simulink model "mrefrobotarm_modified_previous_y_previous_u_previous_ref_pert_2"  (R2018b)
settings: Solver=FixedStepAuto  StartTime=0.0  StopTime=60  RelTol=1e-3  AbsTol=1e-6
undefined symbols (not defined in the file or in its folder): cc, options
libraries: neural x858, simulink x1
(part 14 of 32)

== system mrefrobotarm_modified_previous_y_previous_u_previous_ref_pert_2/m=0 sd=0.01/Layer 3/Delays 1 ==
  "p{3}" : Inport  PortDimensions=30
      mask Display: e = 0.06;c1 = [120 230 180]/255;c2 = ([120 230 180]+0)/(256+128);c3 = ([120 230 180]+128)/(256+128);patch([0 1 1 0],[0 0 1 1],c1);patch([0 1 1 1-e 1-e 0+e],[0 0 1 1-e 0+e 0+e],c2);patch([0 0 1 1-e 0+e 0+e],[0 1 1 1-e 1-e 0+e],c3);plot([0 1 1 0 0],[0 0 1 1 0]);
  mux : Mux  Inputs=1
      mask Display: e = 0.06;c1 = [120 150 230]/255;c2 = ([120 150 230]+0)/383;c3 = ([120 150 230]+128)/383;patch([0 1 1 0],[0 0 1 1],c1);patch([0 1 1 1-e 1-e 0+e],[0 0 1 1-e 0+e 0+e],c2);patch([0 0 1 1-e 0+e 0+e],[0 1 1 1-e 1-e 0+e],c3);plot([0 1 1 0 0],[0 0 1 1 0]);disp('Mux')
  "pd{3,2}" : Outport
      mask Display: e = 0.06;c1 = [120 230 180]/255;c2 = ([120 230 180]+0)/(256+128);c3 = ([120 230 180]+128)/(256+128);patch([0 1 1 0],[0 0 1 1],c1);patch([0 1 1 1-e 1-e 0+e],[0 0 1 1-e 0+e 0+e],c2);patch([0 0 1 1-e 0+e 0+e],[0 1 1 1-e 1-e 0+e],c3);plot([0 1 1 0 0],[0 0 1 1 0]);
  wires:
  "p{3}"/1 -> mux/1
  mux/1 -> "pd{3,2}"/1

== system mrefrobotarm_modified_previous_y_previous_u_previous_ref_pert_2/m=0 sd=0.01/Layer 3/LW{3,2} ==
  "ad{3,2}" : Inport  PortDimensions=30
      mask Display: e = 0.06;c1 = [120 230 180]/255;c2 = ([120 230 180]+0)/(256+128);c3 = ([120 230 180]+128)/(256+128);patch([0 1 1 0],[0 0 1 1],c1);patch([0 1 1 1-e 1-e 0+e],[0 0 1 1-e 0+e 0+e],c2);patch([0 0 1 1-e 0+e 0+e],[0 1 1 1-e 1-e 0+e],c3);plot([0 1 1 0 0],[0 0 1 1 0]);
  "IW{3,2}(1,:)'" : Constant  Value=[0.002729871880378900890484761276866265689022839069366455078125;-0.192793372477307212164987504365853965282440185546875;0.019007002077113754889836627626209519803524017333984375;0.1094735576049869207881926058689714409410953521728515625;-0.0344571917116396064795225129273603670299053192138671875;0.038374723582049762027335049197063199244439601898193359375;-0.271741639414177116318427351870923303067684173583984375;0.0219959957978727548011388392978915362618863582611083984375;0.0298221463111364611109355138296450604684650897979736328125;0.322074127211145644356093953319941647350788116455078125;0.13012962789399995511274710224824957549571990966796875;-0.00019342564852617015642988196333362793666310608386993408203125;0.043919430640314262304091386113213957287371158599853515625;-0.07079981267022698865343244278847123496234416961669921875;-0.039940672099975628450696518711993121542036533355712890625;-0.012214442964989628837013668771760421805083751678466796875;-0.434566982367647181018099900029483251273632049560546875;0.01100983664475223798573377820275709382258355617523193359375;0.013295194727414715030189285016604117117822170257568359375;0.00943231564172179563765308074607673916034400463104248046875;0.016511274981058310373782660462893545627593994140625;0.0083808882427890731003916613417459302581846714019775390625;-0.06728233732539042055709188616674509830772876739501953125;-0.0070167449523096288299672806942908209748566150665283203125;0.1945359442269654903778786092516384087502956390380859375;-0.10981910726153108759373111524837440811097621917724609375;-0.0295376597637224402870259609699132852256298065185546875;0.10283307654067570802158826381855760701000690460205078125;0.059639466058088001776393838326839613728225231170654296875;0.042842060625088405900751098442924558185040950775146484375]
      mask Display: e = 0.06;c1 = [120 150 230]/255;c2 = ([120 150 230]+0)/383;c3 = ([120 150 230]+128)/383;patch([0 1 1 0],[0 0 1 1],c1);patch([0 1 1 1-e 1-e 0+e],[0 0 1 1-e 0+e 0+e],c2);patch([0 0 1 1-e 0+e 0+e],[0 1 1 1-e 1-e 0+e],c3);plot([0 1 1 0 0],[0 0 1 1 0]);disp('weights');
  Mux : Mux  Inputs=1
      mask Display: e = 0.06;c1 = [120 150 230]/255;c2 = ([120 150 230]+0)/383;c3 = ([120 150 230]+128)/383;patch([0 1 1 0],[0 0 1 1],c1);patch([0 1 1 1-e 1-e 0+e],[0 0 1 1-e 0+e 0+e],c2);patch([0 0 1 1-e 0+e 0+e],[0 1 1 1-e 1-e 0+e],c3);plot([0 1 1 0 0],[0 0 1 1 0]);disp('Mux');
  dotprod1 : neural/Weight Functions/dotprod
  "lz{3,2}" : Outport
      mask Display: e = 0.06;c1 = [120 230 180]/255;c2 = ([120 230 180]+0)/(256+128);c3 = ([120 230 180]+128)/(256+128);patch([0 1 1 0],[0 0 1 1],c1);patch([0 1 1 1-e 1-e 0+e],[0 0 1 1-e 0+e 0+e],c2);patch([0 0 1 1-e 0+e 0+e],[0 1 1 1-e 1-e 0+e],c3);plot([0 1 1 0 0],[0 0 1 1 0]);
  wires:
  "IW{3,2}(1,:)'"/1 -> dotprod1/1
  "ad{3,2}"/1 -> dotprod1/2
  dotprod1/1 -> Mux/1
  Mux/1 -> "lz{3,2}"/1

== system mrefrobotarm_modified_previous_y_previous_u_previous_ref_pert_2/m=0 sd=0.1/Layer 1/Delays 1 ==
  "p{1}" : Inport  PortDimensions=10
      mask Display: e = 0.06;c1 = [120 230 180]/255;c2 = ([120 230 180]+0)/(256+128);c3 = ([120 230 180]+128)/(256+128);patch([0 1 1 0],[0 0 1 1],c1);patch([0 1 1 1-e 1-e 0+e],[0 0 1 1-e 0+e 0+e],c2);patch([0 0 1 1-e 0+e 0+e],[0 1 1 1-e 1-e 0+e],c3);plot([0 1 1 0 0],[0 0 1 1 0]);
  mux : Mux  Inputs=1
      mask Display: e = 0.06;c1 = [120 150 230]/255;c2 = ([120 150 230]+0)/383;c3 = ([120 150 230]+128)/383;patch([0 1 1 0],[0 0 1 1],c1);patch([0 1 1 1-e 1-e 0+e],[0 0 1 1-e 0+e 0+e],c2);patch([0 0 1 1-e 0+e 0+e],[0 1 1 1-e 1-e 0+e],c3);plot([0 1 1 0 0],[0 0 1 1 0]);disp('Mux')
  "pd{1,1}" : Outport
      mask Display: e = 0.06;c1 = [120 230 180]/255;c2 = ([120 230 180]+0)/(256+128);c3 = ([120 230 180]+128)/(256+128);patch([0 1 1 0],[0 0 1 1],c1);patch([0 1 1 1-e 1-e 0+e],[0 0 1 1-e 0+e 0+e],c2);patch([0 0 1 1-e 0+e 0+e],[0 1 1 1-e 1-e 0+e],c3);plot([0 1 1 0 0],[0 0 1 1 0]);
  wires:
  "p{1}"/1 -> mux/1
  mux/1 -> "pd{1,1}"/1

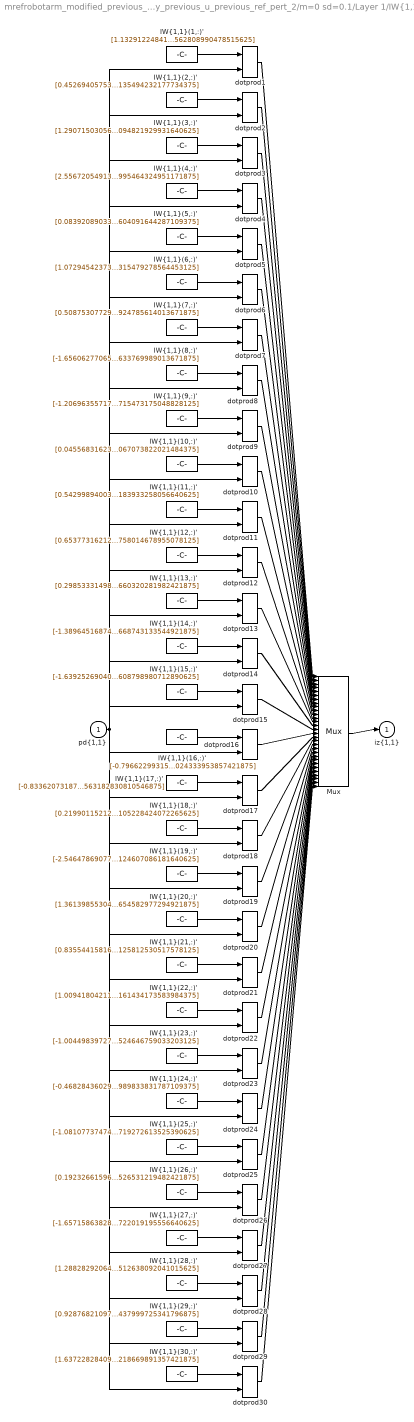
== system mrefrobotarm_modified_previous_y_previous_u_previous_ref_pert_2/m=0 sd=0.1/Layer 1/IW{1,1} ==
  "pd{1,1}" : Inport  PortDimensions=10
      mask Display: e = 0.06;c1 = [120 230 180]/255;c2 = ([120 230 180]+0)/(256+128);c3 = ([120 230 180]+128)/(256+128);patch([0 1 1 0],[0 0 1 1],c1);patch([0 1 1 1-e 1-e 0+e],[0 0 1 1-e 0+e 0+e],c2);patch([0 0 1 1-e 0+e 0+e],[0 1 1 1-e 1-e 0+e],c3);plot([0 1 1 0 0],[0 0 1 1 0]);
  "IW{1,1}(1,:)'" : Constant  Value=[1.132912248415559819392228746437467634677886962890625;-1.66311380994488278162179994978941977024078369140625;1.6836569926662872109801583064836449921131134033203125;-0.72192220583688004875710930718923918902873992919921875;0.1893688932828194448898528889912995509803295135498046875;-0.72187706282018548886725284319254569709300994873046875;-0.244996356013791827255232647075899876654148101806640625;-0.8003255307394396833586824868689291179180145263671875;0.85920037690395700824552704943926073610782623291015625;0.703707694441091380355146611691452562808990478515625]
      mask Display: e = 0.06;c1 = [120 150 230]/255;c2 = ([120 150 230]+0)/383;c3 = ([120 150 230]+128)/383;patch([0 1 1 0],[0 0 1 1],c1);patch([0 1 1 1-e 1-e 0+e],[0 0 1 1-e 0+e 0+e],c2);patch([0 0 1 1-e 0+e 0+e],[0 1 1 1-e 1-e 0+e],c3);plot([0 1 1 0 0],[0 0 1 1 0]);disp('Weights');
  "IW{1,1}(10,:)'" : Constant  Value=[0.04556831623344419213150757741459528915584087371826171875;-1.20856356098407413668383014737628400325775146484375;1.09655271159517742063371770200319588184356689453125;-1.2020275654665344422511452648905105888843536376953125;0.5891689284456680386625748724327422678470611572265625;-0.66781797039911106050880107432021759450435638427734375;0.92909816953891921631480954602011479437351226806640625;0.6734856783720146733429601226816885173320770263671875;-1.280385468531718640150529608945362269878387451171875;-1.3714212414356283797900459830998443067073822021484375]
      mask Display: e = 0.06;c1 = [120 150 230]/255;c2 = ([120 150 230]+0)/383;c3 = ([120 150 230]+128)/383;patch([0 1 1 0],[0 0 1 1],c1);patch([0 1 1 1-e 1-e 0+e],[0 0 1 1-e 0+e 0+e],c2);patch([0 0 1 1-e 0+e 0+e],[0 1 1 1-e 1-e 0+e],c3);plot([0 1 1 0 0],[0 0 1 1 0]);disp('Weights');
  "IW{1,1}(11,:)'" : Constant  Value=[0.5429989400329431337155483561218716204166412353515625;-1.3726786698952084808666995741077698767185211181640625;1.3447843857882892937283259016112424433231353759765625;0.06077100221745439234677377271509612910449504852294921875;0.14702327534578907286544335875078104436397552490234375;-0.9247467487885092651822560583241283893585205078125;1.214941057310911620703564040013588964939117431640625;0.51782811970024644754317932893172837793827056884765625;-0.5071720855890766710416528439964167773723602294921875;-0.84188455536436068715744340806850232183933258056640625]
      mask Display: e = 0.06;c1 = [120 150 230]/255;c2 = ([120 150 230]+0)/383;c3 = ([120 150 230]+128)/383;patch([0 1 1 0],[0 0 1 1],c1);patch([0 1 1 1-e 1-e 0+e],[0 0 1 1-e 0+e 0+e],c2);patch([0 0 1 1-e 0+e 0+e],[0 1 1 1-e 1-e 0+e],c3);plot([0 1 1 0 0],[0 0 1 1 0]);disp('Weights');
  "IW{1,1}(12,:)'" : Constant  Value=[0.6537731621292317552018857895745895802974700927734375;-0.6724403750684089242639629446784965693950653076171875;0.09800014716142928239417386748755234293639659881591796875;-0.0101106387101103749326380665252145263366401195526123046875;0.62476345499575847153295171665376983582973480224609375;-0.98464332271399535034817063205991871654987335205078125;0.29504906959603782734546939536812715232372283935546875;0.08629470772053095262155153477579005993902683258056640625;0.1016581340376631892308267879343475215137004852294921875;-0.63732167330842337538143738129292614758014678955078125]
      mask Display: e = 0.06;c1 = [120 150 230]/255;c2 = ([120 150 230]+0)/383;c3 = ([120 150 230]+128)/383;patch([0 1 1 0],[0 0 1 1],c1);patch([0 1 1 1-e 1-e 0+e],[0 0 1 1-e 0+e 0+e],c2);patch([0 0 1 1-e 0+e 0+e],[0 1 1 1-e 1-e 0+e],c3);plot([0 1 1 0 0],[0 0 1 1 0]);disp('Weights');
  "IW{1,1}(13,:)'" : Constant  Value=[0.29853331498265378574075157303013838827610015869140625;0.10168476545711895020485115992414648644626140594482421875;-0.478832017503906637312383054450037889182567596435546875;-0.345363443456295604594430415090755559504032135009765625;-0.365240575198647998700351990919443778693675994873046875;0.261408879776874325528979170485399663448333740234375;-0.126917798724279384803281800486729480326175689697265625;0.386500317068572074585830478099524043500423431396484375;0.813840320292881447272748118848539888858795166015625;-0.061249010278340447477329888670283253304660320281982421875]
      mask Display: e = 0.06;c1 = [120 150 230]/255;c2 = ([120 150 230]+0)/383;c3 = ([120 150 230]+128)/383;patch([0 1 1 0],[0 0 1 1],c1);patch([0 1 1 1-e 1-e 0+e],[0 0 1 1-e 0+e 0+e],c2);patch([0 0 1 1-e 0+e 0+e],[0 1 1 1-e 1-e 0+e],c3);plot([0 1 1 0 0],[0 0 1 1 0]);disp('Weights');
  "IW{1,1}(14,:)'" : Constant  Value=[-1.3896451687481945480584499819087795913219451904296875;2.15814199825849328817639616318047046661376953125;-1.2683298149542012733803630908369086682796478271484375;-0.11411191741998884252584645082606584765017032623291015625;-0.3155450540943876003296963972388766705989837646484375;0.1251853453557625339698233801755122840404510498046875;-0.00517304141358565679198466824573188205249607563018798828125;-0.64415172505282669579429466466535814106464385986328125;-0.64015313391352479666096542132436297833919525146484375;-0.259011561693888558988163595131481997668743133544921875]
      mask Display: e = 0.06;c1 = [120 150 230]/255;c2 = ([120 150 230]+0)/383;c3 = ([120 150 230]+128)/383;patch([0 1 1 0],[0 0 1 1],c1);patch([0 1 1 1-e 1-e 0+e],[0 0 1 1-e 0+e 0+e],c2);patch([0 0 1 1-e 0+e 0+e],[0 1 1 1-e 1-e 0+e],c3);plot([0 1 1 0 0],[0 0 1 1 0]);disp('Weights');
  "IW{1,1}(15,:)'" : Constant  Value=[-1.639252690409584101161044600303284823894500732421875;0.1935096092033950776478690158910467289388179779052734375;-0.5283754126046869004085237975232303142547607421875;0.57440826056501481655658380987006239593029022216796875;-0.229176783911712311780917161740944720804691314697265625;-1.46447525110886811461341494577936828136444091796875;0.65274531773674382417738115691463463008403778076171875;-0.50645703110697659621308730493183247745037078857421875;-1.0052356537245736856078792698099277913570404052734375;0.48612188066297401523030430325889028608798980712890625]
      mask Display: e = 0.06;c1 = [120 150 230]/255;c2 = ([120 150 230]+0)/383;c3 = ([120 150 230]+128)/383;patch([0 1 1 0],[0 0 1 1],c1);patch([0 1 1 1-e 1-e 0+e],[0 0 1 1-e 0+e 0+e],c2);patch([0 0 1 1-e 0+e 0+e],[0 1 1 1-e 1-e 0+e],c3);plot([0 1 1 0 0],[0 0 1 1 0]);disp('Weights');
  "IW{1,1}(16,:)'" : Constant  Value=[-0.79662299315886742068215653489460237324237823486328125;1.84598954255209957153738287161104381084442138671875;-0.94463712346467065827937403810210525989532470703125;-0.3956089994371831952690854450338520109653472900390625;-0.78376068618349925554156243379111401736736297607421875;-0.38177670775292316118765256760525517165660858154296875;0.61861305262131438542638761646230705082416534423828125;0.020921357743258151007381684394204057753086090087890625;0.4311848034144407648682317812927067279815673828125;-0.1757544230567029408529577949593658559024333953857421875]
      mask Display: e = 0.06;c1 = [120 150 230]/255;c2 = ([120 150 230]+0)/383;c3 = ([120 150 230]+128)/383;patch([0 1 1 0],[0 0 1 1],c1);patch([0 1 1 1-e 1-e 0+e],[0 0 1 1-e 0+e 0+e],c2);patch([0 0 1 1-e 0+e 0+e],[0 1 1 1-e 1-e 0+e],c3);plot([0 1 1 0 0],[0 0 1 1 0]);disp('Weights');
  "IW{1,1}(17,:)'" : Constant  Value=[-0.8336207318746462480163472719141282141208648681640625;0.72618402235620649332048515134374611079692840576171875;-0.53036297580617819402704071762855164706707000732421875;0.64140942781517551463110748954932205379009246826171875;-0.0221842617501962803550075165048838243819773197174072265625;-0.024558325479927707590821484018306364305317401885986328125;0.29991464523139754749792018628795631229877471923828125;0.16921995587321048137852130821556784212589263916015625;-0.90896451623632634753136017025099135935306549072265625;-0.1841664914636124972258102161504211835563182830810546875]
      mask Display: e = 0.06;c1 = [120 150 230]/255;c2 = ([120 150 230]+0)/383;c3 = ([120 150 230]+128)/383;patch([0 1 1 0],[0 0 1 1],c1);patch([0 1 1 1-e 1-e 0+e],[0 0 1 1-e 0+e 0+e],c2);patch([0 0 1 1-e 0+e 0+e],[0 1 1 1-e 1-e 0+e],c3);plot([0 1 1 0 0],[0 0 1 1 0]);disp('Weights');
  "IW{1,1}(18,:)'" : Constant  Value=[0.219901152121808662887048058109940029680728912353515625;-0.09076825686005864091132622206714586354792118072509765625;-0.339186564269195633958275948316440917551517486572265625;-0.502276581787442832904844181030057370662689208984375;-0.413214937935847126393440476022078655660152435302734375;0.406702355871940646192541635173256509006023406982421875;0.015662906329028440655104503775874036364257335662841796875;-0.5416305832111605322864988920628093183040618896484375;0.314207839020848311850642176068504340946674346923828125;0.021790223956706523955606513709426508285105228424072265625]
      mask Display: e = 0.06;c1 = [120 150 230]/255;c2 = ([120 150 230]+0)/383;c3 = ([120 150 230]+128)/383;patch([0 1 1 0],[0 0 1 1],c1);patch([0 1 1 1-e 1-e 0+e],[0 0 1 1-e 0+e 0+e],c2);patch([0 0 1 1-e 0+e 0+e],[0 1 1 1-e 1-e 0+e],c3);plot([0 1 1 0 0],[0 0 1 1 0]);disp('Weights');
  "IW{1,1}(19,:)'" : Constant  Value=[-2.54647869077617716726535945781506597995758056640625;2.074022456073995268610588027513585984706878662109375;-1.264725581662340392341548067633993923664093017578125;0.269992056926158074947608156435308046638965606689453125;0.67791205426768907926771134953014552593231201171875;1.08945288321787092655767992255277931690216064453125;-0.225879558387034384825398092289105989038944244384765625;-0.8743718013102685926440926778013817965984344482421875;1.313495208741327413548560798517428338527679443359375;0.88931998964906144866660042680450715124607086181640625]
      mask Display: e = 0.06;c1 = [120 150 230]/255;c2 = ([120 150 230]+0)/383;c3 = ([120 150 230]+128)/383;patch([0 1 1 0],[0 0 1 1],c1);patch([0 1 1 1-e 1-e 0+e],[0 0 1 1-e 0+e 0+e],c2);patch([0 0 1 1-e 0+e 0+e],[0 1 1 1-e 1-e 0+e],c3);plot([0 1 1 0 0],[0 0 1 1 0]);disp('Weights');
  "IW{1,1}(2,:)'" : Constant  Value=[0.45269405753099623002100315716234035789966583251953125;-1.3819854543589837891914839929086156189441680908203125;1.4394656881736762610302093889913521707057952880859375;-0.498626309305983339559276146246702410280704498291015625;-0.414204872178560890016996154372463934123516082763671875;1.55952109847031028522224005428142845630645751953125;-0.56120044368516330823837279240251518785953521728515625;-0.281840967673469833254529248733888380229473114013671875;3.50820378995669113209032730082981288433074951171875;2.044493088024915916633972301497124135494232177734375]
      mask Display: e = 0.06;c1 = [120 150 230]/255;c2 = ([120 150 230]+0)/383;c3 = ([120 150 230]+128)/383;patch([0 1 1 0],[0 0 1 1],c1);patch([0 1 1 1-e 1-e 0+e],[0 0 1 1-e 0+e 0+e],c2);patch([0 0 1 1-e 0+e 0+e],[0 1 1 1-e 1-e 0+e],c3);plot([0 1 1 0 0],[0 0 1 1 0]);disp('Weights');
  "IW{1,1}(20,:)'" : Constant  Value=[1.361398553041379244632480549626052379608154296875;-1.3859070894705352028353217974654398858547210693359375;-0.400969251454327435535418544532149098813533782958984375;-0.427897979455180876851017046647029928863048553466796875;0.63437067973309779755908266452024690806865692138671875;0.334528713373865083102742801202111877501010894775390625;0.05397557593578884704843545705443830229341983795166015625;0.13660549295664325963883811709820292890071868896484375;1.049795083463204381502009709947742521762847900390625;-0.0200764131524870208245214797670996631495654582977294921875]
      mask Display: e = 0.06;c1 = [120 150 230]/255;c2 = ([120 150 230]+0)/383;c3 = ([120 150 230]+128)/383;patch([0 1 1 0],[0 0 1 1],c1);patch([0 1 1 1-e 1-e 0+e],[0 0 1 1-e 0+e 0+e],c2);patch([0 0 1 1-e 0+e 0+e],[0 1 1 1-e 1-e 0+e],c3);plot([0 1 1 0 0],[0 0 1 1 0]);disp('Weights');
  "IW{1,1}(21,:)'" : Constant  Value=[0.83554415816043192677398110390640795230865478515625;-0.75667157664683060147581272758543491363525390625;-0.05035462838145922381816177448854432441294193267822265625;-0.186509261977637230689452962906216271221637725830078125;0.1779164267290028467183304883292294107377529144287109375;-0.16737486559107284112002389520057477056980133056640625;-0.043842380630178291733844986310941749252378940582275390625;0.30516299405469571315308030534652061760425567626953125;-1.527210479319259572861255946918390691280364990234375;-0.5785736861187509294524033975903876125812530517578125]
      mask Display: e = 0.06;c1 = [120 150 230]/255;c2 = ([120 150 230]+0)/383;c3 = ([120 150 230]+128)/383;patch([0 1 1 0],[0 0 1 1],c1);patch([0 1 1 1-e 1-e 0+e],[0 0 1 1-e 0+e 0+e],c2);patch([0 0 1 1-e 0+e 0+e],[0 1 1 1-e 1-e 0+e],c3);plot([0 1 1 0 0],[0 0 1 1 0]);disp('Weights');
  "IW{1,1}(22,:)'" : Constant  Value=[1.00941804211583718853262325865216553211212158203125;-1.2261900889778554191167359022074379026889801025390625;0.120851782045483469030244805253460071980953216552734375;0.32676568345732548426241237393696792423725128173828125;-0.52634117539310398825591619242914021015167236328125;1.1012958159960113402320303066517226397991180419921875;-0.5060253977059598895493763848207890987396240234375;-0.39813348380348656530003381703863851726055145263671875;1.8147553018736901631058344719349406659603118896484375;1.4870405850798051883288053431897424161434173583984375]
      mask Display: e = 0.06;c1 = [120 150 230]/255;c2 = ([120 150 230]+0)/383;c3 = ([120 150 230]+128)/383;patch([0 1 1 0],[0 0 1 1],c1);patch([0 1 1 1-e 1-e 0+e],[0 0 1 1-e 0+e 0+e],c2);patch([0 0 1 1-e 0+e 0+e],[0 1 1 1-e 1-e 0+e],c3);plot([0 1 1 0 0],[0 0 1 1 0]);disp('Weights');
  "IW{1,1}(23,:)'" : Constant  Value=[-1.0044983972705108232759130260092206299304962158203125;0.1873298225454137211354321834733127616345882415771484375;-0.54804213617540142866602081994642503559589385986328125;-0.70042673178915515475040365345194004476070404052734375;-0.023415375354162000498536855275233392603695392608642578125;-0.95501032317440992525092724463320337235927581787109375;1.0022110698728763367171268328092992305755615234375;-0.76991655197060937521058576749055646359920501708984375;-1.02462948914607299144563512527383863925933837890625;-1.4760810948051397151203900648397393524646759033203125]
      mask Display: e = 0.06;c1 = [120 150 230]/255;c2 = ([120 150 230]+0)/383;c3 = ([120 150 230]+128)/383;patch([0 1 1 0],[0 0 1 1],c1);patch([0 1 1 1-e 1-e 0+e],[0 0 1 1-e 0+e 0+e],c2);patch([0 0 1 1-e 0+e 0+e],[0 1 1 1-e 1-e 0+e],c3);plot([0 1 1 0 0],[0 0 1 1 0]);disp('Weights');
  "IW{1,1}(24,:)'" : Constant  Value=[-0.468284360290036671958802116932929493486881256103515625;1.0621707027343048057588248411775566637516021728515625;-0.91950497784860119043770509961177594959735870361328125;0.050729086990261358647291700663117808289825916290283203125;0.09401277611720904037184709522989578545093536376953125;-0.5526691859768873005265277242870070040225982666015625;0.6698966360936118302760178266908042132854461669921875;-0.1567729090403978398082784906364395283162593841552734375;0.264933900169632863264013167281518690288066864013671875;-0.447551825822690485523480674601159989833831787109375]
      mask Display: e = 0.06;c1 = [120 150 230]/255;c2 = ([120 150 230]+0)/383;c3 = ([120 150 230]+128)/383;patch([0 1 1 0],[0 0 1 1],c1);patch([0 1 1 1-e 1-e 0+e],[0 0 1 1-e 0+e 0+e],c2);patch([0 0 1 1-e 0+e 0+e],[0 1 1 1-e 1-e 0+e],c3);plot([0 1 1 0 0],[0 0 1 1 0]);disp('Weights');
  "IW{1,1}(25,:)'" : Constant  Value=[-1.081077374740320617974020933615975081920623779296875;0.64279083661811375893790909685776568949222564697265625;-0.267842395764306850924896252763574011623859405517578125;0.7450897607842363878916103203664533793926239013671875;0.82627356030284893062543005726183764636516571044921875;-0.39195769077825470816378583549521863460540771484375;-0.202015501963519417127912447540438733994960784912109375;0.89916101439714213316989344093599356710910797119140625;-0.8301541281567679231301326581160537898540496826171875;-0.416799917133972963600996308741741813719272613525390625]
      mask Display: e = 0.06;c1 = [120 150 230]/255;c2 = ([120 150 230]+0)/383;c3 = ([120 150 230]+128)/383;patch([0 1 1 0],[0 0 1 1],c1);patch([0 1 1 1-e 1-e 0+e],[0 0 1 1-e 0+e 0+e],c2);patch([0 0 1 1-e 0+e 0+e],[0 1 1 1-e 1-e 0+e],c3);plot([0 1 1 0 0],[0 0 1 1 0]);disp('Weights');
  "IW{1,1}(26,:)'" : Constant  Value=[0.1923266159612029568837243687084992416203022003173828125;-0.80992252631693961717473939643241465091705322265625;-0.14493676196781934972790395477204583585262298583984375;-1.1229707457292572581053491376223973929882049560546875;-0.54252404045220148365302748061367310583591461181640625;-1.06886334868473031889379853964783251285552978515625;0.9948315499383790783127778922789730131626129150390625;0.152465655384979414943558140294044278562068939208984375;-0.68998166028190721643653660066775046288967132568359375;-1.4428166074457855483359480786020867526531219482421875]
      mask Display: e = 0.06;c1 = [120 150 230]/255;c2 = ([120 150 230]+0)/383;c3 = ([120 150 230]+128)/383;patch([0 1 1 0],[0 0 1 1],c1);patch([0 1 1 1-e 1-e 0+e],[0 0 1 1-e 0+e 0+e],c2);patch([0 0 1 1-e 0+e 0+e],[0 1 1 1-e 1-e 0+e],c3);plot([0 1 1 0 0],[0 0 1 1 0]);disp('Weights');
  "IW{1,1}(27,:)'" : Constant  Value=[-1.6571586382832157458011579365120269358158111572265625;2.86298728904135391104546215501613914966583251953125;-0.7213543770211312544660131607088260352611541748046875;0.301232704656333172277271614802884869277477264404296875;-0.016745756818622899164683559547484037466347217559814453125;-0.82008705446743979106116739785647951066493988037109375;0.65578457676010992738468985407962463796138763427734375;-0.68340853893493924697821739755454473197460174560546875;0.1911644525940358885218728346444549970328807830810546875;-0.0288623922702351022595568252882003434933722019195556640625]
      mask Display: e = 0.06;c1 = [120 150 230]/255;c2 = ([120 150 230]+0)/383;c3 = ([120 150 230]+128)/383;patch([0 1 1 0],[0 0 1 1],c1);patch([0 1 1 1-e 1-e 0+e],[0 0 1 1-e 0+e 0+e],c2);patch([0 0 1 1-e 0+e 0+e],[0 1 1 1-e 1-e 0+e],c3);plot([0 1 1 0 0],[0 0 1 1 0]);disp('Weights');
  "IW{1,1}(28,:)'" : Constant  Value=[1.2882829206406238853332979488186538219451904296875;-0.62425953029952607753472193508059717714786529541015625;-0.59190041246323155110786728982930071651935577392578125;0.53647381032516161525336428894661366939544677734375;0.42978817559882898091672132068197242915630340576171875;0.70153054187913921335706390891573391854763031005859375;-0.458324045413930847292505177392740733921527862548828125;-0.50252223793030947884830084149143658578395843505859375;-0.91259450157277643977948855535942129790782928466796875;-0.130631405538267186816625553547055460512638092041015625]
      mask Display: e = 0.06;c1 = [120 150 230]/255;c2 = ([120 150 230]+0)/383;c3 = ([120 150 230]+128)/383;patch([0 1 1 0],[0 0 1 1],c1);patch([0 1 1 1-e 1-e 0+e],[0 0 1 1-e 0+e 0+e],c2);patch([0 0 1 1-e 0+e 0+e],[0 1 1 1-e 1-e 0+e],c3);plot([0 1 1 0 0],[0 0 1 1 0]);disp('Weights');
  "IW{1,1}(29,:)'" : Constant  Value=[0.92876821097719874931186723188147880136966705322265625;-0.316191487680865190856849267220241017639636993408203125;-0.9663850736922203754630800176528282463550567626953125;-0.68849439879813878473413524261559359729290008544921875;-0.429687888689719910129127811160287819802761077880859375;0.289887888189278408734850245309644378721714019775390625;1.278858531308505686041598892188630998134613037109375;-0.8698389651444429215843001657049171626567840576171875;1.0468948855574324863226820525596849620342254638671875;-0.1539409925282792801493059187123435549437999725341796875]
      mask Display: e = 0.06;c1 = [120 150 230]/255;c2 = ([120 150 230]+0)/383;c3 = ([120 150 230]+128)/383;patch([0 1 1 0],[0 0 1 1],c1);patch([0 1 1 1-e 1-e 0+e],[0 0 1 1-e 0+e 0+e],c2);patch([0 0 1 1-e 0+e 0+e],[0 1 1 1-e 1-e 0+e],c3);plot([0 1 1 0 0],[0 0 1 1 0]);disp('Weights');
  "IW{1,1}(3,:)'" : Constant  Value=[1.2907150305671650780681147807626985013484954833984375;-1.5769416133466929164086423043045215308666229248046875;-0.66001303824557966404285025419085286557674407958984375;0.52837771369532327003781801977311260998249053955078125;0.521070941990531277809850507765077054500579833984375;-0.74814857171303950078566913362010382115840911865234375;1.02852301966715931058615751680918037891387939453125;-0.1321655342391363507914547881227917969226837158203125;-0.456989775756285798724576352469739504158496856689453125;-0.6231284026776793272262011669226922094821929931640625]
      mask Display: e = 0.06;c1 = [120 150 230]/255;c2 = ([120 150 230]+0)/383;c3 = ([120 150 230]+128)/383;patch([0 1 1 0],[0 0 1 1],c1);patch([0 1 1 1-e 1-e 0+e],[0 0 1 1-e 0+e 0+e],c2);patch([0 0 1 1-e 0+e 0+e],[0 1 1 1-e 1-e 0+e],c3);plot([0 1 1 0 0],[0 0 1 1 0]);disp('Weights');
  "IW{1,1}(30,:)'" : Constant  Value=[1.637228284090687768781435806886292994022369384765625;-1.846953752864070708028521039523184299468994140625;0.6806049332873114199315978112281300127506256103515625;-0.56541885127706914548895156258367933332920074462890625;-1.2699089669929273238579980898066423833370208740234375;1.86689761180617797009517744299955666065216064453125;-1.1232513546886908617494782447465695440769195556640625;0.1453674639014009006832139903053757734596729278564453125;1.0509840057341672814317234951886348426342010498046875;1.505179218361568427297925154562108218669891357421875]
      mask Display: e = 0.06;c1 = [120 150 230]/255;c2 = ([120 150 230]+0)/383;c3 = ([120 150 230]+128)/383;patch([0 1 1 0],[0 0 1 1],c1);patch([0 1 1 1-e 1-e 0+e],[0 0 1 1-e 0+e 0+e],c2);patch([0 0 1 1-e 0+e 0+e],[0 1 1 1-e 1-e 0+e],c3);plot([0 1 1 0 0],[0 0 1 1 0]);disp('Weights');
  "IW{1,1}(4,:)'" : Constant  Value=[2.556720549135189202161200228147208690643310546875;-3.258857965265137490717961554764769971370697021484375;1.1401735662930827519545573522918857634067535400390625;-0.527964829625254150613500314648263156414031982421875;1.9440738356444582368709461661637760698795318603515625;-0.7482336793844714950552088339463807642459869384765625;-0.3204906509866918273843339193263091146945953369140625;1.06815648950187647159282278153114020824432373046875;-0.0890878366209650607299153080020914785563945770263671875;-0.98332734514651221058301189259509555995464324951171875]
      mask Display: e = 0.06;c1 = [120 150 230]/255;c2 = ([120 150 230]+0)/383;c3 = ([120 150 230]+128)/383;patch([0 1 1 0],[0 0 1 1],c1);patch([0 1 1 1-e 1-e 0+e],[0 0 1 1-e 0+e 0+e],c2);patch([0 0 1 1-e 0+e 0+e],[0 1 1 1-e 1-e 0+e],c3);plot([0 1 1 0 0],[0 0 1 1 0]);disp('Weights');
  "IW{1,1}(5,:)'" : Constant  Value=[0.08392089033110028406525771060842089354991912841796875;-0.01076518165151564392079119869549685972742736339569091796875;-0.76431051909334024596631707026972435414791107177734375;0.005445241138962057976524722135991396498866379261016845703125;-1.113896888451066491398933067102916538715362548828125;1.1829549197050621689442095885169692337512969970703125;-0.1452638359721234173616011275953496806323528289794921875;0.09505325241205352104767456467016017995774745941162109375;0.824643225782639266441265135654248297214508056640625;1.148108113835907939659364274120889604091644287109375]
      mask Display: e = 0.06;c1 = [120 150 230]/255;c2 = ([120 150 230]+0)/383;c3 = ([120 150 230]+128)/383;patch([0 1 1 0],[0 0 1 1],c1);patch([0 1 1 1-e 1-e 0+e],[0 0 1 1-e 0+e 0+e],c2);patch([0 0 1 1-e 0+e 0+e],[0 1 1 1-e 1-e 0+e],c3);plot([0 1 1 0 0],[0 0 1 1 0]);disp('Weights');
  "IW{1,1}(6,:)'" : Constant  Value=[1.0729454237326871979263387402170337736606597900390625;-1.02897733435734739515510227647610008716583251953125;0.529513108661344933381087685120292007923126220703125;-0.160761617828738045954395374792511574923992156982421875;-0.255155535700625157868870473976130597293376922607421875;-0.4693729374857118497033070525503717362880706787109375;0.92985584320082781406568983584293164312839508056640625;-0.203429108007346759467992569625494070351123809814453125;0.0677569643726999848443171003964380361139774322509765625;-0.5436491628863440173091703400132246315479278564453125]
      mask Display: e = 0.06;c1 = [120 150 230]/255;c2 = ([120 150 230]+0)/383;c3 = ([120 150 230]+128)/383;patch([0 1 1 0],[0 0 1 1],c1);patch([0 1 1 1-e 1-e 0+e],[0 0 1 1-e 0+e 0+e],c2);patch([0 0 1 1-e 0+e 0+e],[0 1 1 1-e 1-e 0+e],c3);plot([0 1 1 0 0],[0 0 1 1 0]);disp('Weights');
  "IW{1,1}(7,:)'" : Constant  Value=[0.5087530772928250399900207412429153919219970703125;-0.72275590797490962824412008558283559978008270263671875;0.98703592833260522798610736572300083935260772705078125;0.0745257436909177173323115539460559375584125518798828125;-0.515275994488835209494936862029135227203369140625;0.408520690147010867576682358048856258392333984375;0.7049744986580306349566171775222755968570709228515625;-0.5187749998269481910284639525343663990497589111328125;-0.655588975122619377344790336792357265949249267578125;-1.192263238986935647290010820142924785614013671875]
      mask Display: e = 0.06;c1 = [120 150 230]/255;c2 = ([120 150 230]+0)/383;c3 = ([120 150 230]+128)/383;patch([0 1 1 0],[0 0 1 1],c1);patch([0 1 1 1-e 1-e 0+e],[0 0 1 1-e 0+e 0+e],c2);patch([0 0 1 1-e 0+e 0+e],[0 1 1 1-e 1-e 0+e],c3);plot([0 1 1 0 0],[0 0 1 1 0]);disp('Weights');
  "IW{1,1}(8,:)'" : Constant  Value=[-1.656062770656069549346511848852969706058502197265625;1.0799485487971907105020363815128803253173828125;1.07643846673486809351061310735531151294708251953125;-0.11388515890106561123662487489127670414745807647705078125;0.34417213396941293002129214073647744953632354736328125;-0.035461693978427459572611013527421164326369762420654296875;-1.3084703437418314653228890165337361395359039306640625;0.1805781658817567081332100542567786760628223419189453125;1.492291368578742893902244759374298155307769775390625;1.223695843846154929224212537519633769989013671875]
      mask Display: e = 0.06;c1 = [120 150 230]/255;c2 = ([120 150 230]+0)/383;c3 = ([120 150 230]+128)/383;patch([0 1 1 0],[0 0 1 1],c1);patch([0 1 1 1-e 1-e 0+e],[0 0 1 1-e 0+e 0+e],c2);patch([0 0 1 1-e 0+e 0+e],[0 1 1 1-e 1-e 0+e],c3);plot([0 1 1 0 0],[0 0 1 1 0]);disp('Weights');
  "IW{1,1}(9,:)'" : Constant  Value=[-1.2069635571783063898720911311102099716663360595703125;-0.1954715592676647684111657099492731504142284393310546875;2.2208001581531267021318853949196636676788330078125;-0.56222673478999263263489183373167179524898529052734375;1.2816598991110985661379118027980439364910125732421875;1.4310647588806173491349227333557792007923126220703125;-2.554919380782112892092072797822766005992889404296875;0.2336960307259200730900516873589367605745792388916015625;0.63656718069432993711842527773114852607250213623046875;1.1105605139442176199082723542232997715473175048828125]
      mask Display: e = 0.06;c1 = [120 150 230]/255;c2 = ([120 150 230]+0)/383;c3 = ([120 150 230]+128)/383;patch([0 1 1 0],[0 0 1 1],c1);patch([0 1 1 1-e 1-e 0+e],[0 0 1 1-e 0+e 0+e],c2);patch([0 0 1 1-e 0+e 0+e],[0 1 1 1-e 1-e 0+e],c3);plot([0 1 1 0 0],[0 0 1 1 0]);disp('Weights');
  Mux : Mux  Inputs=30
      mask Display: e = 0.06;c1 = [120 150 230]/255;c2 = ([120 150 230]+0)/383;c3 = ([120 150 230]+128)/383;patch([0 1 1 0],[0 0 1 1],c1);patch([0 1 1 1-e 1-e 0+e],[0 0 1 1-e 0+e 0+e],c2);patch([0 0 1 1-e 0+e 0+e],[0 1 1 1-e 1-e 0+e],c3);plot([0 1 1 0 0],[0 0 1 1 0]);disp('Mux');
  dotprod{1..30} (30 alike) : neural/Weight Functions/dotprod
  "iz{1,1}" : Outport
      mask Display: e = 0.06;c1 = [120 230 180]/255;c2 = ([120 230 180]+0)/(256+128);c3 = ([120 230 180]+128)/(256+128);patch([0 1 1 0],[0 0 1 1],c1);patch([0 1 1 1-e 1-e 0+e],[0 0 1 1-e 0+e 0+e],c2);patch([0 0 1 1-e 0+e 0+e],[0 1 1 1-e 1-e 0+e],c3);plot([0 1 1 0 0],[0 0 1 1 0]);
  wires:
  "IW{1,1}(1,:)'"/1 -> dotprod1/1
  "pd{1,1}"/1 -> dotprod1/2, dotprod2/2, dotprod3/2, dotprod4/2, dotprod5/2, dotprod6/2, dotprod7/2, dotprod8/2, dotprod9/2, dotprod10/2, dotprod11/2, dotprod12/2, dotprod13/2, dotprod14/2, dotprod15/2, dotprod16/2, dotprod17/2, dotprod18/2, dotprod19/2, dotprod20/2, dotprod21/2, dotprod22/2, dotprod23/2, dotprod24/2, dotprod25/2, dotprod26/2, dotprod27/2, dotprod28/2, dotprod29/2, dotprod30/2
  dotprod1/1 -> Mux/1
  "IW{1,1}(2,:)'"/1 -> dotprod2/1
  dotprod2/1 -> Mux/2
  "IW{1,1}(3,:)'"/1 -> dotprod3/1
  dotprod3/1 -> Mux/3
  "IW{1,1}(4,:)'"/1 -> dotprod4/1
  dotprod4/1 -> Mux/4
  "IW{1,1}(5,:)'"/1 -> dotprod5/1
  dotprod5/1 -> Mux/5
  "IW{1,1}(6,:)'"/1 -> dotprod6/1
  dotprod6/1 -> Mux/6
  "IW{1,1}(7,:)'"/1 -> dotprod7/1
  dotprod7/1 -> Mux/7
  "IW{1,1}(8,:)'"/1 -> dotprod8/1
  dotprod8/1 -> Mux/8
  "IW{1,1}(9,:)'"/1 -> dotprod9/1
  dotprod9/1 -> Mux/9
  "IW{1,1}(10,:)'"/1 -> dotprod10/1
  dotprod10/1 -> Mux/10
  "IW{1,1}(11,:)'"/1 -> dotprod11/1
  dotprod11/1 -> Mux/11
  "IW{1,1}(12,:)'"/1 -> dotprod12/1
  dotprod12/1 -> Mux/12
  "IW{1,1}(13,:)'"/1 -> dotprod13/1
  dotprod13/1 -> Mux/13
  "IW{1,1}(14,:)'"/1 -> dotprod14/1
  dotprod14/1 -> Mux/14
  "IW{1,1}(15,:)'"/1 -> dotprod15/1
  dotprod15/1 -> Mux/15
  "IW{1,1}(16,:)'"/1 -> dotprod16/1
  dotprod16/1 -> Mux/16
  "IW{1,1}(17,:)'"/1 -> dotprod17/1
  dotprod17/1 -> Mux/17
  "IW{1,1}(18,:)'"/1 -> dotprod18/1
  dotprod18/1 -> Mux/18
  "IW{1,1}(19,:)'"/1 -> dotprod19/1
  dotprod19/1 -> Mux/19
  "IW{1,1}(20,:)'"/1 -> dotprod20/1
  dotprod20/1 -> Mux/20
  "IW{1,1}(21,:)'"/1 -> dotprod21/1
  dotprod21/1 -> Mux/21
  "IW{1,1}(22,:)'"/1 -> dotprod22/1
  dotprod22/1 -> Mux/22
  "IW{1,1}(23,:)'"/1 -> dotprod23/1
  dotprod23/1 -> Mux/23
  "IW{1,1}(24,:)'"/1 -> dotprod24/1
  dotprod24/1 -> Mux/24
  "IW{1,1}(25,:)'"/1 -> dotprod25/1
  dotprod25/1 -> Mux/25
  "IW{1,1}(26,:)'"/1 -> dotprod26/1
  dotprod26/1 -> Mux/26
  "IW{1,1}(27,:)'"/1 -> dotprod27/1
  dotprod27/1 -> Mux/27
  "IW{1,1}(28,:)'"/1 -> dotprod28/1
  dotprod28/1 -> Mux/28
  "IW{1,1}(29,:)'"/1 -> dotprod29/1
  dotprod29/1 -> Mux/29
  "IW{1,1}(30,:)'"/1 -> dotprod30/1
  dotprod30/1 -> Mux/30
  Mux/1 -> "iz{1,1}"/1

== system mrefrobotarm_modified_previous_y_previous_u_previous_ref_pert_2/m=0 sd=0.1/Layer 2/Delays 1 ==
  "p{2}" : Inport  PortDimensions=30
      mask Display: e = 0.06;c1 = [120 230 180]/255;c2 = ([120 230 180]+0)/(256+128);c3 = ([120 230 180]+128)/(256+128);patch([0 1 1 0],[0 0 1 1],c1);patch([0 1 1 1-e 1-e 0+e],[0 0 1 1-e 0+e 0+e],c2);patch([0 0 1 1-e 0+e 0+e],[0 1 1 1-e 1-e 0+e],c3);plot([0 1 1 0 0],[0 0 1 1 0]);
  mux : Mux  Inputs=1
      mask Display: e = 0.06;c1 = [120 150 230]/255;c2 = ([120 150 230]+0)/383;c3 = ([120 150 230]+128)/383;patch([0 1 1 0],[0 0 1 1],c1);patch([0 1 1 1-e 1-e 0+e],[0 0 1 1-e 0+e 0+e],c2);patch([0 0 1 1-e 0+e 0+e],[0 1 1 1-e 1-e 0+e],c3);plot([0 1 1 0 0],[0 0 1 1 0]);disp('Mux')
  "pd{2,1}" : Outport
      mask Display: e = 0.06;c1 = [120 230 180]/255;c2 = ([120 230 180]+0)/(256+128);c3 = ([120 230 180]+128)/(256+128);patch([0 1 1 0],[0 0 1 1],c1);patch([0 1 1 1-e 1-e 0+e],[0 0 1 1-e 0+e 0+e],c2);patch([0 0 1 1-e 0+e 0+e],[0 1 1 1-e 1-e 0+e],c3);plot([0 1 1 0 0],[0 0 1 1 0]);
  wires:
  "p{2}"/1 -> mux/1
  mux/1 -> "pd{2,1}"/1
